simulink model "Task3b"  (R2015a)
settings: Solver=ode3  StartTime=0.0  StopTime=20  FixedStep=0.001  RelTol=1e-3
values from neighbouring files (symbols this model uses):
  a1 = 0.1    [slip.m]
  amp = 1    [slip.m]
  amp1 = 1    [slip.m]
  B = 0.1    [slip.m]
  c = 1    [slip.m]
  C = 40    [slip.m]
  freq1 = 10    [slip.m]
  g = 9.81    [slip.m]
  I = 1.4    [slip.m]
  k1 = 1500    [slip.m]
  m = 250    [slip.m]
  Mu_Max = 0.003    [slip.m]
  p1 = 1000    [slip.m]
  R = 0.275    [slip.m]
  v_0 = 120/3.6    (= 33.3333333333)    [slip.m]
  w_0 = v_0/R    (= 121.212121212)    [slip.m]
undefined symbols (not defined in the file or in its folder): B1
libraries: simulink x2
settings Model: Creator=DMori  LastModifiedBy=DMori
settings DataIOCC: LimitDataPoints=off

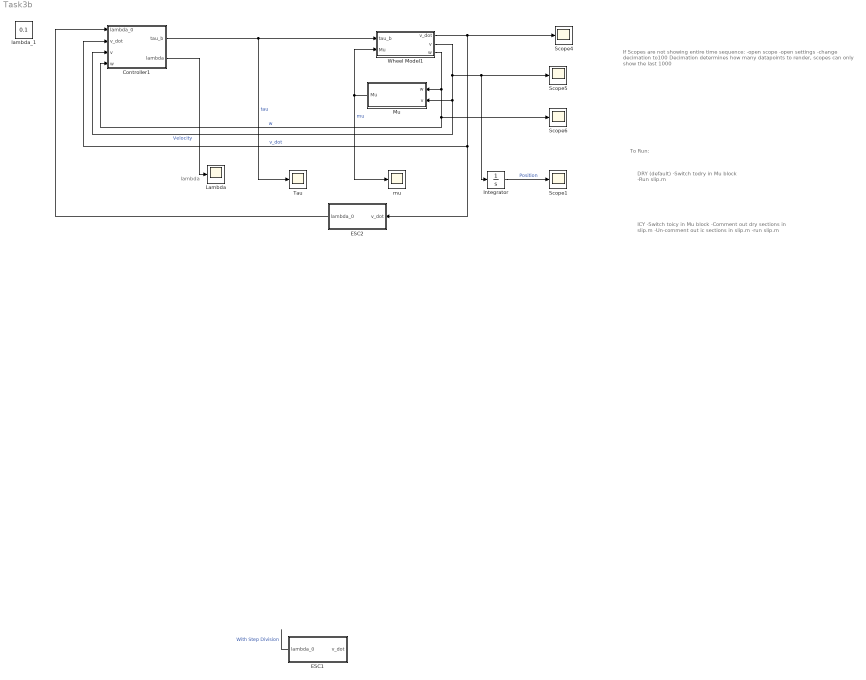
== system Task3b ==
  note: lambda
  note: If Scopes are not showing entire time sequence:
      | -open scope
      | -open settings
      | -change decimation to100
      | Decimation determines how many
      | datapoints to render, scopes can only show the last 1000
  note: DRY (default)
      | -Switch todry in Mu block
      | -Run slip.m
  note: ICY
      | -Switch toicy in Mu block
      | -Comment out dry sections in slip.m
      | -Un-comment out ic sections in slip.m
      | -run slip.m
  note: To Run:
  Controller1 : Subsystem
  ESC1 : Subsystem
  ESC2 : Subsystem
  Integrator : Integrator
  Lambda : Scope
      settings: ShowLegends=on  TimeRange=40  YMin=-0.05  YMax=0.2  SaveName=ScopeData5  Decimation=10
  Mu : Subsystem
  Scope{1,4..6} (4 alike) : Scope
      Scope1 settings: ShowLegends=on  TimeRange=40  YMin=-0.05  YMax=0.2  SaveName=ScopeData8  Decimation=10
      Scope4 settings: ShowLegends=on  TimeRange=40  YMin=-0.05  YMax=0.2  SaveName=ScopeData2  Decimation=10
      Scope5 settings: ShowLegends=on  TimeRange=40  YMin=-0.05  YMax=0.2  SaveName=ScopeData3  Decimation=10
      Scope6 settings: ShowLegends=on  TimeRange=40  YMin=-0.05  YMax=0.2  SaveName=ScopeData4  Decimation=10
  Tau : Scope
      settings: ShowLegends=on  TimeRange=40  YMin=-0.05  YMax=0.2  Decimation=10
  Wheel Model1 : Subsystem
  lambda_1 : Constant  Value=0.1
  mu : Scope
      settings: ShowLegends=on  TimeRange=40  YMin=-0.05  YMax=0.2  Decimation=10
  wires:
  Wheel Model1/1(v_dot) -> Scope4/1, ESC2/1(v_dot), Controller1/2(v_dot)  "v_dot"
  Controller1/1(tau_b) -> Tau/1, Wheel Model1/1(tau_b)  "tau"
  Wheel Model1/3(w) -> Controller1/4(w), Scope6/1, Mu/1(w)  "w"
  Wheel Model1/2(v) -> Controller1/3(v), Mu/2(v), Integrator/1, Scope5/1  "Velocity"
  Mu/1(Mu) -> Wheel Model1/2(Mu), mu/1  "mu"
  Controller1/2(lambda) -> Lambda/1
  ESC2/1(lambda_0) -> Controller1/1(lambda_0)
  ESC1/1(lambda_0) -> ?  "With Step Division"
  Integrator/1 -> Scope1/1  "Position"

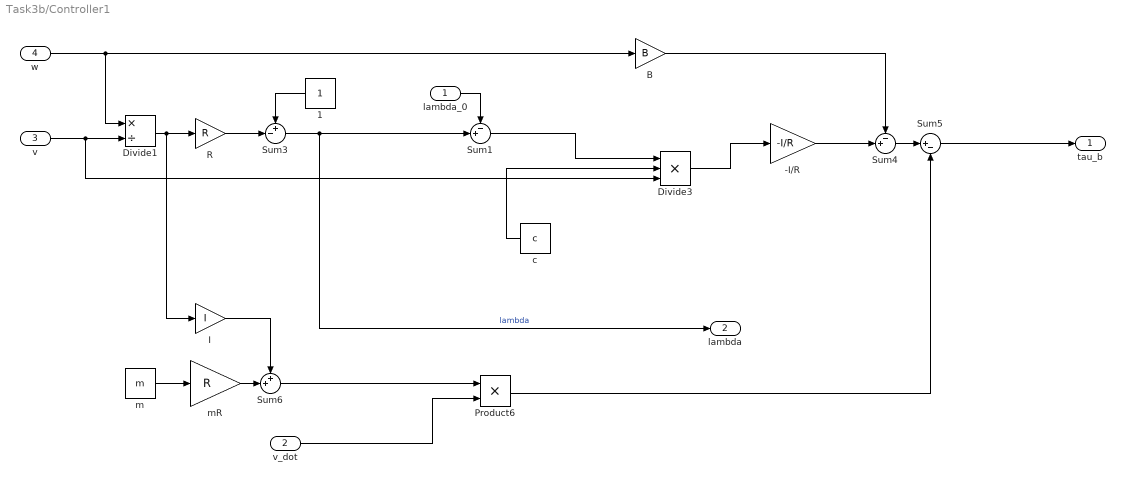
== system Task3b/Controller1 ==
  lambda_0 : Inport
  v_dot : Inport  Port=2
  v : Inport  Port=3
  w : Inport  Port=4
  -I/R : Gain  Gain=-I/R
  1 : Constant
  B : Gain  Gain=B
  Divide1 : Product  Inputs=*/
  Divide3 : Product  Inputs=***
  I : Gain  Gain=I
  Product6 : Product
  R : Gain  Gain=R
  Sum1 : Sum  Inputs=-+|
  Sum3 : Sum  Inputs=+-|
  Sum4 : Sum  Inputs=-+|
  Sum5 : Sum  Inputs=|+-
  Sum6 : Sum  Inputs=++|
  c : Constant  Value=c
  m : Constant  Value=m
  mR : Gain  Gain=R
  tau_b : Outport
  lambda : Outport  Port=2
  wires:
  Sum1/1 -> Divide3/1
  m/1 -> mR/1
  Divide1/1 -> I/1, R/1
  1/1 -> Sum3/1
  R/1 -> Sum3/2
  w/1 -> Divide1/1, B/1
  v/1 -> Divide3/3, Divide1/2
  Divide3/1 -> -I/R/1
  -I/R/1 -> Sum4/2
  B/1 -> Sum4/1
  mR/1 -> Sum6/2
  I/1 -> Sum6/1
  Sum6/1 -> Product6/1
  Sum4/1 -> Sum5/1
  Product6/1 -> Sum5/2
  v_dot/1 -> Product6/2
  lambda_0/1 -> Sum1/1
  Sum5/1 -> tau_b/1
  Sum3/1 -> lambda/1, Sum1/2  "lambda"
  c/1 -> Divide3/2

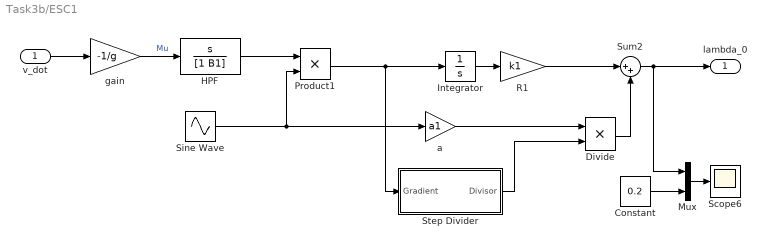
== system Task3b/ESC1 ==
  v_dot : Inport
  Constant : Constant  Value=0.2
  Divide : Product  Inputs=**
  HPF : TransferFcn  Numerator=[1 0]  Denominator=[1 B1]
  Integrator : Integrator
  Mux : Mux  Inputs=2
  Product1 : Product
  R1 : Gain  Gain=k1
  Scope6 : Scope
      settings: TimeRange=40  YMin=0  YMax=0.2  SaveName=ScopeData31  Decimation=100
  Sine Wave : Sin  Amplitude=amp  Frequency=freq1  SampleTime=0
  Step Divider : Subsystem
  Sum2 : Sum  Inputs=|++
  a : Gain  Gain=a1
  gain : Gain  Gain=-1/g
  lambda_0 : Outport
  wires:
  Integrator/1 -> R1/1
  R1/1 -> Sum2/1
  Sine Wave/1 -> a/1, Product1/2
  Product1/1 -> Step Divider/1(Gradient), Integrator/1
  v_dot/1 -> gain/1
  gain/1 -> HPF/1  "Mu"
  HPF/1 -> Product1/1
  Mux/1 -> Scope6/1
  Sum2/1 -> Mux/1, lambda_0/1
  a/1 -> Divide/1
  Divide/1 -> Sum2/2
  Step Divider/1(Divisor) -> Divide/2
  Constant/1 -> Mux/2

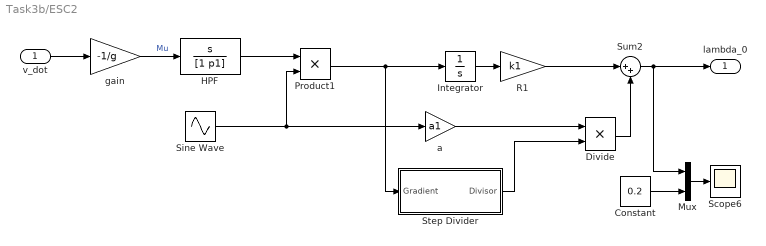
== system Task3b/ESC2 ==
  v_dot : Inport
  Constant : Constant  Value=0.2
  Divide : Product  Inputs=**
  HPF : TransferFcn  Numerator=[1 0]  Denominator=[1 p1]
  Integrator : Integrator
  Mux : Mux  Inputs=2
  Product1 : Product
  R1 : Gain  Gain=k1
  Scope6 : Scope
      settings: TimeRange=40  YMin=0  YMax=0.2  SaveName=ScopeData31  Decimation=100
  Sine Wave : Sin  Amplitude=amp1  Frequency=freq1  SampleTime=0
  Step Divider : Subsystem
  Sum2 : Sum  Inputs=|++
  a : Gain  Gain=a1
  gain : Gain  Gain=-1/g
  lambda_0 : Outport
  wires:
  Integrator/1 -> R1/1
  R1/1 -> Sum2/1
  Sine Wave/1 -> a/1, Product1/2
  Product1/1 -> Step Divider/1(Gradient), Integrator/1
  v_dot/1 -> gain/1
  gain/1 -> HPF/1  "Mu"
  HPF/1 -> Product1/1
  Mux/1 -> Scope6/1
  Sum2/1 -> Mux/1, lambda_0/1
  a/1 -> Divide/1
  Divide/1 -> Sum2/2
  Step Divider/1(Divisor) -> Divide/2
  Constant/1 -> Mux/2

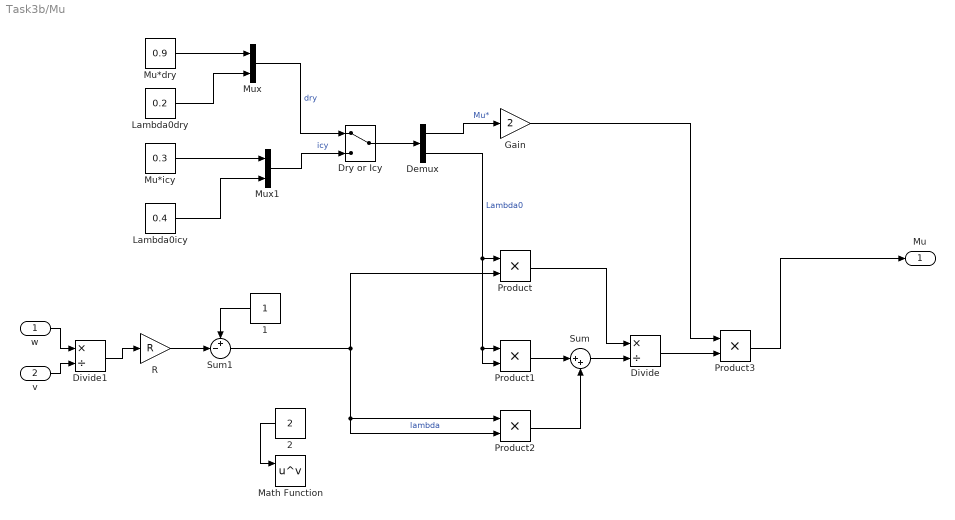
== system Task3b/Mu ==
  w : Inport
  v : Inport  Port=2
  1 : Constant
  2 : Constant  Value=2
  Demux : Demux  Outputs=2
  Divide : Product  Inputs=*/
  Divide1 : Product  Inputs=*/
  Dry or Icy : ManualSwitch
  Gain : Gain  Gain=2
  Lambda0dry : Constant  Value=0.2
  Lambda0icy : Constant  Value=0.4
  Math Function : Math  Operator=pow  SaturateOnIntegerOverflow=on
  Mu*dry : Constant  Value=0.9
  Mu*icy : Constant  Value=0.3
  Mux : Mux  Inputs=2
  Mux1 : Mux  Inputs=2
  Product{,1..3} (4 alike) : Product
  R : Gain  Gain=R
  Sum : Sum  Inputs=|++
  Sum1 : Sum  Inputs=+-|
  Mu : Outport
  wires:
  Lambda0dry/1 -> Mux/2
  Mu*dry/1 -> Mux/1
  Mux/1 -> Dry or Icy/1  "dry"
  Mux1/1 -> Dry or Icy/2  "icy"
  Mu*icy/1 -> Mux1/1
  Lambda0icy/1 -> Mux1/2
  Dry or Icy/1 -> Demux/1
  Demux/1 -> Gain/1  "Mu*"
  Demux/2 -> Product1/2, Product1/1, Product/1  "Lambda0"
  Sum1/1 -> Product2/2, Product2/1, Product/2  "lambda"
  Product/1 -> Divide/1
  Product2/1 -> Sum/2
  Product1/1 -> Sum/1
  Sum/1 -> Divide/2
  Divide/1 -> Product3/2
  Gain/1 -> Product3/1
  Product3/1 -> Mu/1
  Divide1/1 -> R/1
  1/1 -> Sum1/1
  R/1 -> Sum1/2
  w/1 -> Divide1/1
  v/1 -> Divide1/2
  2/1 -> Math Function/1

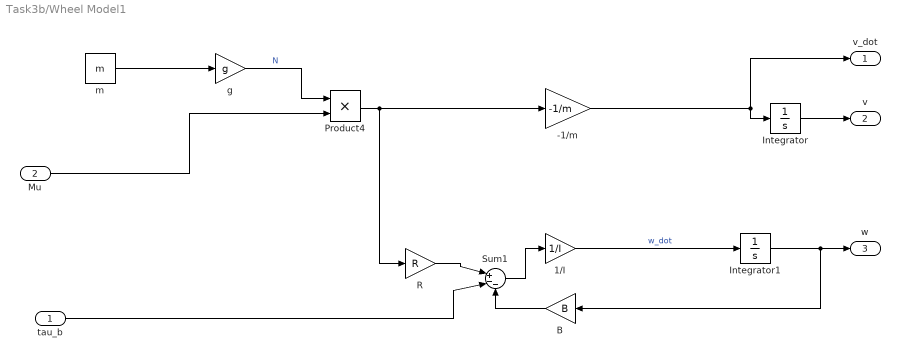
== system Task3b/Wheel Model1 ==
  tau_b : Inport
  Mu : Inport  Port=2
  -1/m : Gain  Gain=-1/m
  1/I : Gain  Gain=1/I
  B : Gain  Gain=B
  Integrator : Integrator  InitialCondition=v_0
  Integrator1 : Integrator  InitialCondition=w_0
  Product4 : Product
  R : Gain  Gain=R
  Sum1 : Sum  Inputs=|+--
  g : Gain  Gain=g
  m : Constant  Value=m
  v_dot : Outport
  v : Outport  Port=2
  w : Outport  Port=3
  wires:
  g/1 -> Product4/1  "N"
  Mu/1 -> Product4/2
  m/1 -> g/1
  Integrator/1 -> v/1
  Integrator1/1 -> B/1, w/1
  Product4/1 -> -1/m/1, R/1
  B/1 -> Sum1/3
  1/I/1 -> Integrator1/1  "w_dot"
  R/1 -> Sum1/1
  Sum1/1 -> 1/I/1
  tau_b/1 -> Sum1/2
  -1/m/1 -> Integrator/1, v_dot/1

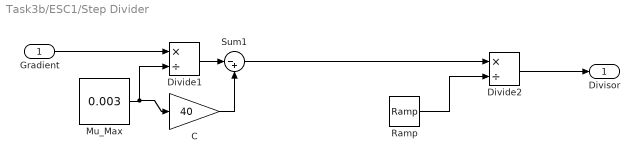
== system Task3b/ESC1/Step Divider ==
  Gradient : Inport
  C : Gain  Gain=40
  Divide1 : Product  Inputs=*/
  Divide2 : Product  Inputs=*/
  Mu_Max : Constant  Value=0.003
  Ramp : simulink/Sources/Ramp  slope=1  start=3  X0=1
  Sum1 : Sum  Inputs=|-+
  Divisor : Outport
  wires:
  Divide1/1 -> Sum1/1
  Mu_Max/1 -> Divide1/2, C/1
  C/1 -> Sum1/2
  Sum1/1 -> Divide2/1
  Ramp/1 -> Divide2/2
  Divide2/1 -> Divisor/1
  Gradient/1 -> Divide1/1

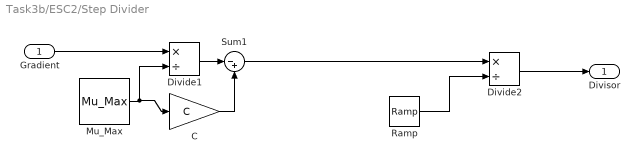
== system Task3b/ESC2/Step Divider ==
  Gradient : Inport
  C : Gain  Gain=C
  Divide1 : Product  Inputs=*/
  Divide2 : Product  Inputs=*/
  Mu_Max : Constant  Value=Mu_Max
  Ramp : simulink/Sources/Ramp  slope=1  start=3  X0=1
  Sum1 : Sum  Inputs=|-+
  Divisor : Outport
  wires:
  Divide1/1 -> Sum1/1
  Mu_Max/1 -> Divide1/2, C/1
  C/1 -> Sum1/2
  Sum1/1 -> Divide2/1
  Ramp/1 -> Divide2/2
  Divide2/1 -> Divisor/1
  Gradient/1 -> Divide1/1
